simulink model "ind_trig"  (Simulink 4.00)
settings: Solver=ode45  StartTime=0.0  StopTime=10.0  RelTol=1e-3
libraries: simulink3 x3
settings Model: ConsistencyChecking=warning  BlockReductionOpt=off

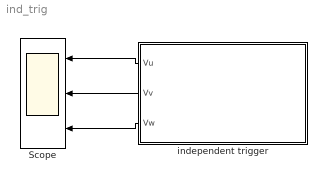
== system ind_trig ==
  Scope : Scope  NumInputPorts=3
      settings: TimeRange=auto  YMin=-5~-5~-5  YMax=5~5~5  SaveToWorkspace=off  SaveName=ScopeData  MaxDataPoints=5000
  independent trigger : Subsystem  Orientation=left  mask{T=1/80}
      mask prompts: T "Time period"
      settings: RTWFcnNameOpts=Auto  RTWFileNameOpts=Auto
  wires:
  independent trigger/1(Vu) -> Scope/1
  independent trigger/2(Vv) -> Scope/2
  independent trigger/3(Vw) -> Scope/3

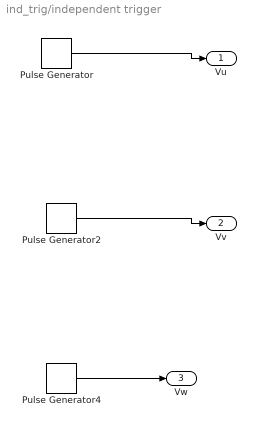
== system ind_trig/independent trigger ==
  Pulse Generator : simulink3/Sources/Pulse Generator  period=T  duty=50  amplitude=1  start=0
  Pulse Generator2 : simulink3/Sources/Pulse Generator  period=T  duty=50  amplitude=1  start=4*T/12
  Pulse Generator4 : simulink3/Sources/Pulse Generator  period=T  duty=50  amplitude=1  start=-4*T/12
  Vu : Outport  Port=1
  Vv : Outport  Port=2
  Vw : Outport  Port=3
  wires:
  Pulse Generator/1 -> Vu/1
  Pulse Generator2/1 -> Vv/1
  Pulse Generator4/1 -> Vw/1
